simulink library "SCR"  (R2025b)
settings: Solver=VariableStepAuto  StartTime=0.0  StopTime=10.0  RelTol=1e-3
libraries: slpidlib x4
settings Model: Creator=Michael  LastModifiedBy=Michael

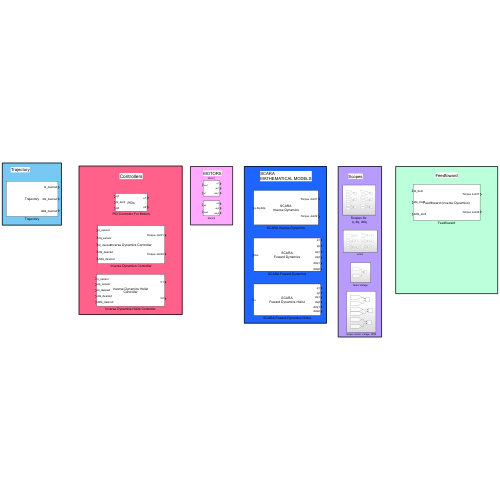
[thumbnail: Simulink's stored preview of the top-level diagram]
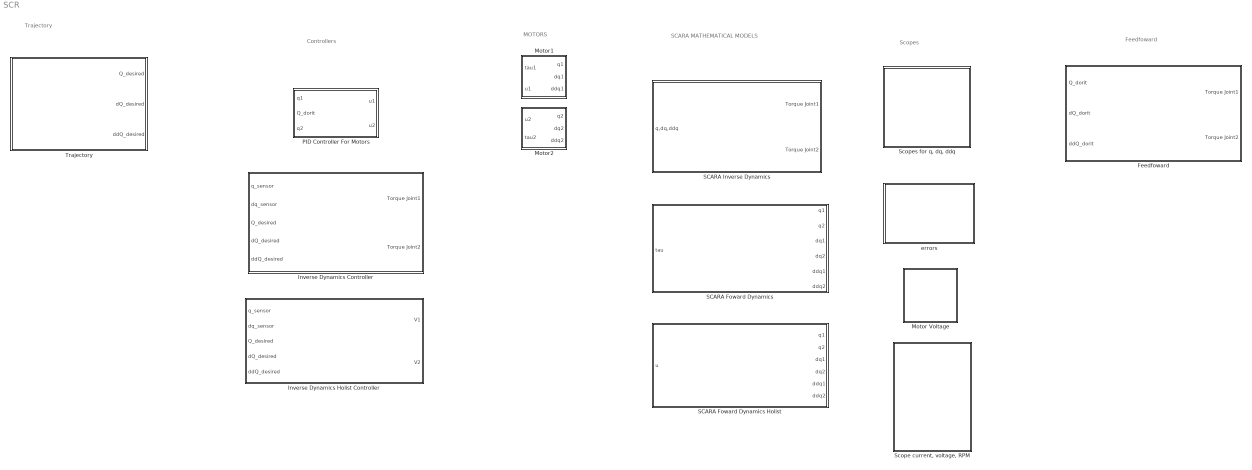
== system SCR ==
  note: MOTORS
  note: SCARA
      | MATHEMATICAL MODELS
  note: Scopes
  note: Trajectory
  note: Controllers
  note: Feedfoward
  Feedfoward : Subsystem
      mask Display: disp("Feedfoward (Inverse Dynamics)")
  Inverse Dynamics Controller : Subsystem
      mask Display: disp("Inverse Dynamics Controller")
  Inverse Dynamics Holist Controller : Subsystem
      mask Display:
      | disp("Inverse Dynamics Holist\n")
      | disp("\nController")
  Motor Voltage : Subsystem
  Motor1 : Subsystem
  Motor2 : Subsystem
  PID Controller For Motors : Subsystem
      mask Display: disp("PIDs")
  SCARA Foward Dynamics : Subsystem
      mask Display:
      | disp("SCARA\n")
      | disp("\nFoward Dynamics")
  SCARA Foward Dynamics Holist : Subsystem
      mask Display:
      | disp("SCARA\n")
      | disp("\nFoward Dynamics Holist")
  SCARA Inverse Dynamics : Subsystem
      mask Display:
      | disp("SCARA\n")
      | disp("\nInverse Dynamics")
  "Scope current, voltage, RPM" : Subsystem
  "Scopes for q, dq, ddq" : Subsystem
  Trajectory : Subsystem
      mask Display: disp("Trajectory")
  errors : Subsystem

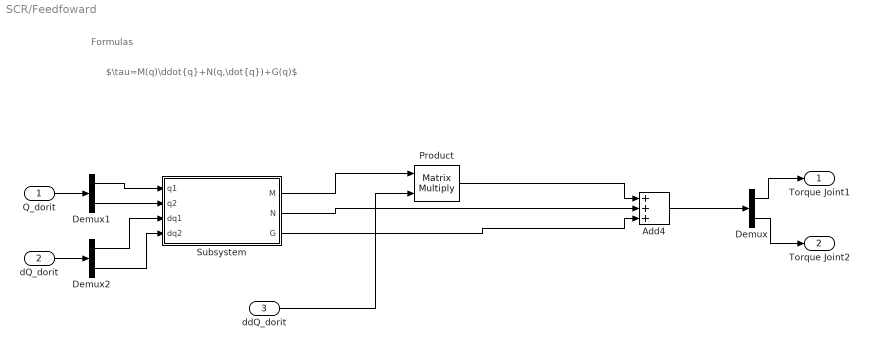
== system SCR/Feedfoward ==
  note: Formulas
  note: $\tau=M(q)\ddot{q}​+N(q,\dot{q})+G(q)$
  Q_dorit : Inport
  dQ_dorit : Inport  Port=2
  ddQ_dorit : Inport  Port=3
  Add4 : Sum  Inputs=+++
  Demux : Demux  Outputs=2
  Demux1 : Demux  Outputs=2
  Demux2 : Demux  Outputs=2
  Product : Product  Multiplication=Matrix(*)
  Subsystem : Subsystem
      mask Display: disp("Tau Components")
  Torque Joint1 : Outport
  Torque Joint2 : Outport  Port=2
  wires:
  Product/1 -> Add4/1
  Add4/1 -> Demux/1
  Demux/2 -> Torque Joint2/1
  Demux/1 -> Torque Joint1/1
  Subsystem/3(G) -> Add4/3
  Subsystem/1(M) -> Product/1
  Subsystem/2(N) -> Add4/2
  Q_dorit/1 -> Demux1/1
  Demux1/1 -> Subsystem/1(q1)
  Demux1/2 -> Subsystem/2(q2)
  dQ_dorit/1 -> Demux2/1
  Demux2/1 -> Subsystem/3(dq1)
  Demux2/2 -> Subsystem/4(dq2)
  ddQ_dorit/1 -> Product/2

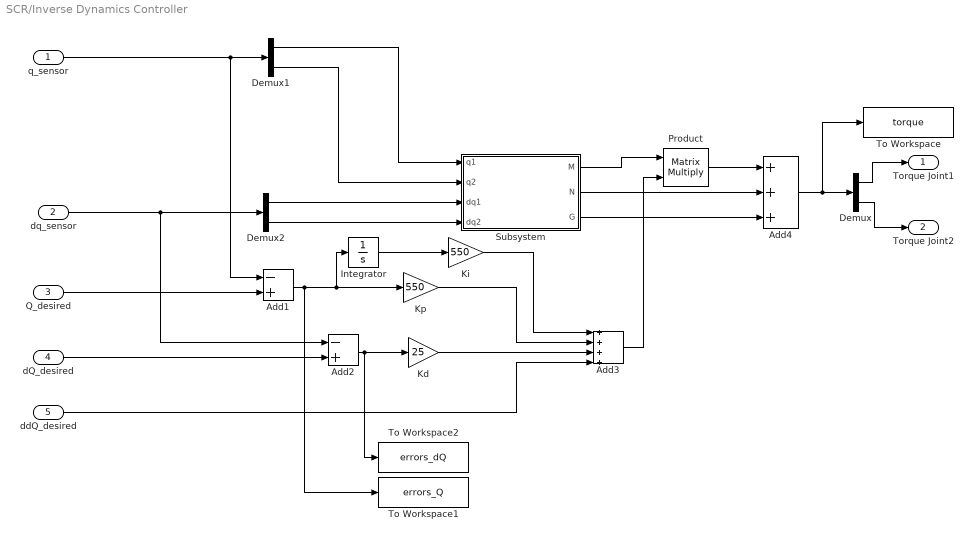
== system SCR/Inverse Dynamics Controller ==
  q_sensor : Inport
  dq_sensor : Inport  Port=2
  Q_desired : Inport  Port=3
  dQ_desired : Inport  Port=4
  ddQ_desired : Inport  Port=5
  Add1 : Sum  Inputs=-+
  Add2 : Sum  Inputs=-+
  Add3 : Sum  Inputs=++++
  Add4 : Sum  Inputs=+++
  Demux : Demux  Outputs=2
  Demux1 : Demux  Outputs=2
  Demux2 : Demux  Outputs=2
  Integrator : Integrator
  Kd : Gain  Gain=25
  Ki : Gain  Gain=550
  Kp : Gain  Gain=550
  Product : Product  Multiplication=Matrix(*)
  Subsystem : Subsystem
      mask Display: disp("Tau Components")
  To Workspace : ToWorkspace  VariableName=torque  SaveFormat=Timeseries  SampleTime=-1
  To Workspace1 : ToWorkspace  VariableName=errors_Q  SaveFormat=Timeseries  SampleTime=-1
  To Workspace2 : ToWorkspace  VariableName=errors_dQ  SaveFormat=Timeseries  SampleTime=-1
  Torque Joint1 : Outport
  Torque Joint2 : Outport  Port=2
  wires:
  Demux1/2 -> Subsystem/2(q2)
  dQ_desired/1 -> Add2/2
  Add1/1 -> Kp/1, Integrator/1, To Workspace1/1
  Add2/1 -> Kd/1, To Workspace2/1
  Add3/1 -> Product/2
  Add4/1 -> To Workspace/1, Demux/1
  Demux/2 -> Torque Joint2/1
  Demux/1 -> Torque Joint1/1
  Q_desired/1 -> Add1/2
  q_sensor/1 -> Add1/1, Demux1/1
  dq_sensor/1 -> Add2/1, Demux2/1
  Subsystem/1(M) -> Product/1
  Demux2/1 -> Subsystem/3(dq1)
  Demux2/2 -> Subsystem/4(dq2)
  Subsystem/2(N) -> Add4/2
  Demux1/1 -> Subsystem/1(q1)
  ddQ_desired/1 -> Add3/4
  Kd/1 -> Add3/3
  Kp/1 -> Add3/2
  Ki/1 -> Add3/1
  Integrator/1 -> Ki/1
  Subsystem/3(G) -> Add4/3
  Product/1 -> Add4/1

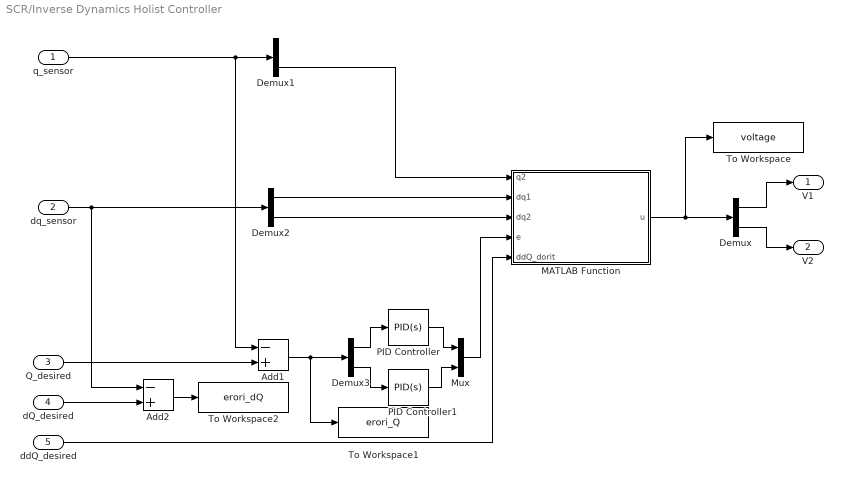
== system SCR/Inverse Dynamics Holist Controller ==
  q_sensor : Inport
  dq_sensor : Inport  Port=2
  Q_desired : Inport  Port=3
  dQ_desired : Inport  Port=4
  ddQ_desired : Inport  Port=5
  Add1 : Sum  Inputs=-+
  Add2 : Sum  Inputs=-+
  Demux{,1..3} (4 alike) : Demux  Outputs=2
  MATLAB Function : MATLAB Function  TreatAsAtomicUnit=on
  Mux : Mux  Inputs=2
  PID Controller : slpidlib/PID Controller  Controller=PID  Form=Parallel  TimeDomain=Continuous-time  UseExternalTs=off  SampleTime=-1  IntegratorMethod=Forward Euler  FilterMethod=Forward Euler  ControllerParametersSource=internal  P=14.7787089689118  I=5.05842239486125  UseKiTs=off  D=9.92816544136059  UseExternalDerivativeSource=off  N=1142.8279760416  UseFilter=on  TunerSelectOption=Transfer Function Based (PID Tuner App)  InitialConditionSource=internal  InitialConditionForIntegrator=0  InitialConditionForFilter=0  DifferentiatorICPrevScaledInput=0  ExternalReset=none  TrackingMode=off  Kt=1  LimitOutput=off  SatLimitsSource=internal  UpperSaturationLimit=0  LowerSaturationLimit=0  LinearizeAsGain=on  AntiWindupMode=none  Kb=1  LimitIntegrator=off  UpperIntegratorSaturationLimit=inf  LowerIntegratorSaturationLimit=-inf  POutMin=[]  POutMax=[]  IOutMin=[]  IOutMax=[]  DOutMin=[]  DOutMax=[]  NOutMin=[]  NOutMax=[]  SumOutMin=[]  SumOutMax=[]  SaturationOutMin=[]  SaturationOutMax=[]  PParamMin=[]  PParamMax=[]  IParamMin=[]  IParamMax=[]  DParamMin=[]  DParamMax=[]  NParamMin=[]  NParamMax=[]  KbParamMin=[]  KbParamMax=[]  KtParamMin=[]  KtParamMax=[]  KbOutMin=[]  KbOutMax=[]  KtOutMin=[]  KtOutMax=[]  IntegratorOutMin=[]  IntegratorOutMax=[]  FilterOutMin=[]  FilterOutMax=[]  SumI1OutMin=[]  SumI1OutMax=[]  SumI2OutMin=[]  SumI2OutMax=[]  SumI3OutMin=[]  SumI3OutMax=[]  SumI4OutMin=[]  SumI4OutMax=[]  SumDOutMin=[]  SumDOutMax=[]  DifferentiatorOutMin=[]  DifferentiatorOutMax=[]  FilterDiffOutCoefMin=[]  FilterDiffOutCoefMax=[]  ReciprocalOutMin=[]  ReciprocalOutMax=[]  SumDenOutMin=[]  SumDenOutMax=[]  SumNumOutMin=[]  SumNumOutMax=[]  DivideOutMin=[]  DivideOutMax=[]  UdiffTsProdOutMin=[]  UdiffTsProdOutMax=[]  NTsProdOutMin=[]  NTsProdOutMax=[]  UintegralTsProdOutMin=[]  UintegralTsProdOutMax=[]  UngainTsProdOutMin=[]  UngainTsProdOutMax=[]  ClampingZeroOutDataTypeStr=Inherit: Inherit via back propagation  ClampingZeroOutMin=[]  ClampingZeroOutMax=[]  FilterDenConstantOutDataTypeStr=Inherit: Inherit via back propagation  FilterDenConstantOutMin=[]  FilterDenConstantOutMax=[]  PCopyOutDataTypeStr=Inherit: Inherit via back propagation  PCopyOutMin=[]  PCopyOutMax=[]  NCopyOutDataTypeStr=Inherit: Inherit via back propagation  NCopyOutMin=[]  NCopyOutMax=[]  IntegratorContinuousStateAttributes=''  IntegratorStateMustResolveToSignalObject=off  IntegratorRTWStateStorageClass=Auto  FilterContinuousStateAttributes=''  FilterStateMustResolveToSignalObject=off  FilterRTWStateStorageClass=Auto  ParallelPVariant=InternalParameters  IdealPVariant=Disabled  IVariant=InternalParameters  DVariant=InternalParameters  IntegratorVariant=Continuous  SatVariant=Disabled  AWVariant=Passthrough  PCopyVariant=Disabled  TRVariant=Disabled  FdbkBlocksVariant=Forward  IdealPFdbkVariant=Disabled  SatFdbkVariant=Disabled  DerivativeFilterVariant=ContFilter  NVariant=InternalParameters  NCopyVariant=Disabled  FilterICVariant=InternalICsFilter  IntegratorICVariant=InternalICs  ExternalResetVariant=Disabled  TRSumVariant=Passthrough  SumFdbkVariant=Disabled  SumVariant=Sum_PID  TsampFilterVariant=InternalTs  TsampNgainVariant=Passthrough  TsampIntegralVariant=Disabled_SignalSpec  ExternalSaturationOutDataTypeStr=Inherit: Same as second input  DerivativeSourceVariant=ErrorSignal  PreIntVariant=InternalPreInt
  PID Controller1 : slpidlib/PID Controller  Controller=PID  Form=Parallel  TimeDomain=Continuous-time  UseExternalTs=off  SampleTime=-1  IntegratorMethod=Forward Euler  FilterMethod=Forward Euler  ControllerParametersSource=internal  P=16.3330424592972  I=6.55014962380407  UseKiTs=off  D=9.91721708236017  UseExternalDerivativeSource=off  N=1142.8279760416  UseFilter=on  TunerSelectOption=Transfer Function Based (PID Tuner App)  InitialConditionSource=internal  InitialConditionForIntegrator=0  InitialConditionForFilter=0  DifferentiatorICPrevScaledInput=0  ExternalReset=none  TrackingMode=off  Kt=1  LimitOutput=off  SatLimitsSource=internal  UpperSaturationLimit=24  LowerSaturationLimit=-24  LinearizeAsGain=on  AntiWindupMode=none  Kb=1  LimitIntegrator=off  UpperIntegratorSaturationLimit=inf  LowerIntegratorSaturationLimit=-inf  POutMin=[]  POutMax=[]  IOutMin=[]  IOutMax=[]  DOutMin=[]  DOutMax=[]  NOutMin=[]  NOutMax=[]  SumOutMin=[]  SumOutMax=[]  SaturationOutMin=[]  SaturationOutMax=[]  PParamMin=[]  PParamMax=[]  IParamMin=[]  IParamMax=[]  DParamMin=[]  DParamMax=[]  NParamMin=[]  NParamMax=[]  KbParamMin=[]  KbParamMax=[]  KtParamMin=[]  KtParamMax=[]  KbOutMin=[]  KbOutMax=[]  KtOutMin=[]  KtOutMax=[]  IntegratorOutMin=[]  IntegratorOutMax=[]  FilterOutMin=[]  FilterOutMax=[]  SumI1OutMin=[]  SumI1OutMax=[]  SumI2OutMin=[]  SumI2OutMax=[]  SumI3OutMin=[]  SumI3OutMax=[]  SumI4OutMin=[]  SumI4OutMax=[]  SumDOutMin=[]  SumDOutMax=[]  DifferentiatorOutMin=[]  DifferentiatorOutMax=[]  FilterDiffOutCoefMin=[]  FilterDiffOutCoefMax=[]  ReciprocalOutMin=[]  ReciprocalOutMax=[]  SumDenOutMin=[]  SumDenOutMax=[]  SumNumOutMin=[]  SumNumOutMax=[]  DivideOutMin=[]  DivideOutMax=[]  UdiffTsProdOutMin=[]  UdiffTsProdOutMax=[]  NTsProdOutMin=[]  NTsProdOutMax=[]  UintegralTsProdOutMin=[]  UintegralTsProdOutMax=[]  UngainTsProdOutMin=[]  UngainTsProdOutMax=[]  ClampingZeroOutDataTypeStr=Inherit: Inherit via back propagation  ClampingZeroOutMin=[]  ClampingZeroOutMax=[]  FilterDenConstantOutDataTypeStr=Inherit: Inherit via back propagation  FilterDenConstantOutMin=[]  FilterDenConstantOutMax=[]  PCopyOutDataTypeStr=Inherit: Inherit via back propagation  PCopyOutMin=[]  PCopyOutMax=[]  NCopyOutDataTypeStr=Inherit: Inherit via back propagation  NCopyOutMin=[]  NCopyOutMax=[]  IntegratorContinuousStateAttributes=''  IntegratorStateMustResolveToSignalObject=off  IntegratorRTWStateStorageClass=Auto  FilterContinuousStateAttributes=''  FilterStateMustResolveToSignalObject=off  FilterRTWStateStorageClass=Auto  ParallelPVariant=InternalParameters  IdealPVariant=Disabled  IVariant=InternalParameters  DVariant=InternalParameters  IntegratorVariant=Continuous  SatVariant=Disabled  AWVariant=Passthrough  PCopyVariant=Disabled  TRVariant=Disabled  FdbkBlocksVariant=Forward  IdealPFdbkVariant=Disabled  SatFdbkVariant=Disabled  DerivativeFilterVariant=ContFilter  NVariant=InternalParameters  NCopyVariant=Disabled  FilterICVariant=InternalICsFilter  IntegratorICVariant=InternalICs  ExternalResetVariant=Disabled  TRSumVariant=Passthrough  SumFdbkVariant=Disabled  SumVariant=Sum_PID  TsampFilterVariant=InternalTs  TsampNgainVariant=Passthrough  TsampIntegralVariant=Disabled_SignalSpec  ExternalSaturationOutDataTypeStr=Inherit: Same as second input  DerivativeSourceVariant=ErrorSignal  PreIntVariant=InternalPreInt
  To Workspace : ToWorkspace  VariableName=voltage  SaveFormat=Timeseries  SampleTime=-1
  To Workspace1 : ToWorkspace  VariableName=erori_Q  SaveFormat=Timeseries  SampleTime=-1
  To Workspace2 : ToWorkspace  VariableName=erori_dQ  SaveFormat=Timeseries  SampleTime=-1
  V1 : Outport
  V2 : Outport  Port=2
  wires:
  Demux2/1 -> MATLAB Function/2(dq1)
  Demux1/2 -> MATLAB Function/1(q2)
  Mux/1 -> MATLAB Function/4(e)
  PID Controller1/1 -> Mux/2
  PID Controller/1 -> Mux/1
  Demux3/2 -> PID Controller1/1
  Demux3/1 -> PID Controller/1
  Add1/1 -> To Workspace1/1, Demux3/1
  MATLAB Function/1(u) -> To Workspace/1, Demux/1
  ddQ_desired/1 -> MATLAB Function/5(ddQ_dorit)
  Demux2/2 -> MATLAB Function/3(dq2)
  dq_sensor/1 -> Add2/1, Demux2/1
  q_sensor/1 -> Demux1/1, Add1/1
  Q_desired/1 -> Add1/2
  Demux/1 -> V1/1
  Demux/2 -> V2/1
  dQ_desired/1 -> Add2/2
  Add2/1 -> To Workspace2/1

== system SCR/Motor Voltage ==
  motorTorques : Scope  NumInputPorts=2
      settings: DataLoggingVariableName=ScopeData6
  wires:
  [u1] -> motorTorques/1
  [u2] -> motorTorques/2

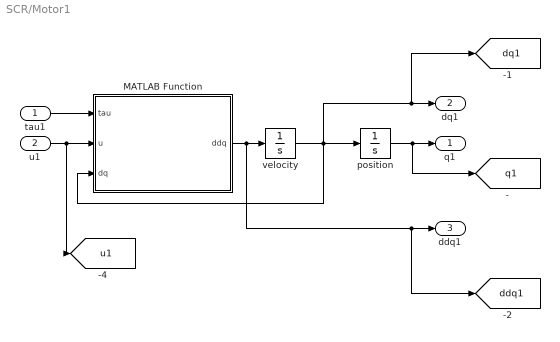
== system SCR/Motor1 ==
  tau1 : Inport
  u1 : Inport  Port=2
  MATLAB Function : MATLAB Function  TreatAsAtomicUnit=on
  position : Integrator
  velocity : Integrator
  q1 : Outport
  dq1 : Outport  Port=2
  ddq1 : Outport  Port=3
  tag scope: ddq1=global, dq1=global, q1=global, u1=global
  wires:
  MATLAB Function/1(ddq) -> [ddq1], ddq1/1, velocity/1
  u1/1 -> [u1], MATLAB Function/2(u)
  tau1/1 -> MATLAB Function/1(tau)
  velocity/1 -> [dq1], dq1/1, MATLAB Function/3(dq), position/1
  position/1 -> [q1], q1/1

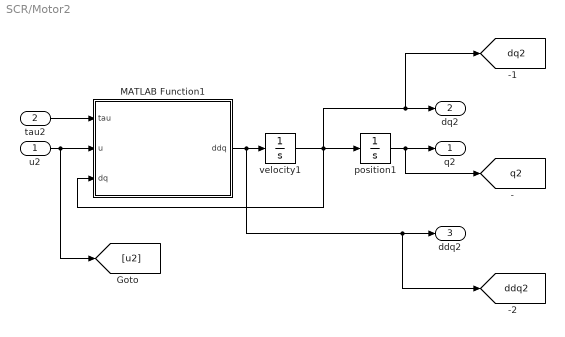
== system SCR/Motor2 ==
  u2 : Inport
  tau2 : Inport  Port=2
  MATLAB Function1 : MATLAB Function  TreatAsAtomicUnit=on
  position1 : Integrator
  velocity1 : Integrator
  q2 : Outport
  dq2 : Outport  Port=2
  ddq2 : Outport  Port=3
  tag scope: ddq2=global, dq2=global, q2=global
  wires:
  MATLAB Function1/1(ddq) -> [ddq2], ddq2/1, velocity1/1
  velocity1/1 -> [dq2], dq2/1, MATLAB Function1/3(dq), position1/1
  tau2/1 -> MATLAB Function1/1(tau)
  position1/1 -> [q2], q2/1
  u2/1 -> [u2], MATLAB Function1/2(u)

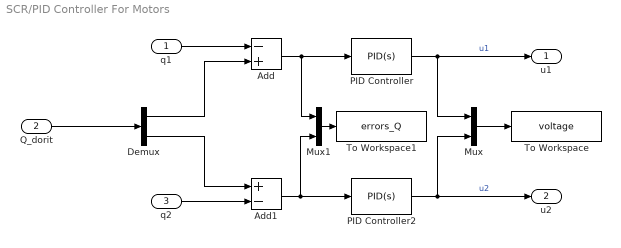
== system SCR/PID Controller For Motors ==
  q1 : Inport
  Q_dorit : Inport  Port=2
  q2 : Inport  Port=3
  Add : Sum  Inputs=-+
  Add1 : Sum  Inputs=+-
  Demux : Demux  Outputs=2
  Mux : Mux  Inputs=2
  Mux1 : Mux  Inputs=2
  PID Controller : slpidlib/PID Controller  Controller=PID  Form=Parallel  TimeDomain=Continuous-time  UseExternalTs=off  SampleTime=-1  IntegratorMethod=Forward Euler  FilterMethod=Forward Euler  ControllerParametersSource=internal  P=17042.9277196606  I=696153.474275857  UseKiTs=off  D=-7.42275649016862  UseExternalDerivativeSource=off  N=2296.03756262702  UseFilter=on  TunerSelectOption=Transfer Function Based (PID Tuner App)  InitialConditionSource=internal  InitialConditionForIntegrator=0  InitialConditionForFilter=0  DifferentiatorICPrevScaledInput=0  ExternalReset=none  TrackingMode=off  Kt=1  LimitOutput=on  SatLimitsSource=internal  UpperSaturationLimit=24  LowerSaturationLimit=-24  LinearizeAsGain=off  AntiWindupMode=clamping  Kb=10  LimitIntegrator=off  UpperIntegratorSaturationLimit=inf  LowerIntegratorSaturationLimit=-inf  POutMin=[]  POutMax=[]  IOutMin=[]  IOutMax=[]  DOutMin=[]  DOutMax=[]  NOutMin=[]  NOutMax=[]  SumOutMin=[]  SumOutMax=[]  SaturationOutMin=[]  SaturationOutMax=[]  PParamMin=[]  PParamMax=[]  IParamMin=[]  IParamMax=[]  DParamMin=[]  DParamMax=[]  NParamMin=[]  NParamMax=[]  KbParamMin=[]  KbParamMax=[]  KtParamMin=[]  KtParamMax=[]  KbOutMin=[]  KbOutMax=[]  KtOutMin=[]  KtOutMax=[]  IntegratorOutMin=[]  IntegratorOutMax=[]  FilterOutMin=[]  FilterOutMax=[]  SumI1OutMin=[]  SumI1OutMax=[]  SumI2OutMin=[]  SumI2OutMax=[]  SumI3OutMin=[]  SumI3OutMax=[]  SumI4OutMin=[]  SumI4OutMax=[]  SumDOutMin=[]  SumDOutMax=[]  DifferentiatorOutMin=[]  DifferentiatorOutMax=[]  FilterDiffOutCoefMin=[]  FilterDiffOutCoefMax=[]  ReciprocalOutMin=[]  ReciprocalOutMax=[]  SumDenOutMin=[]  SumDenOutMax=[]  SumNumOutMin=[]  SumNumOutMax=[]  DivideOutMin=[]  DivideOutMax=[]  UdiffTsProdOutMin=[]  UdiffTsProdOutMax=[]  NTsProdOutMin=[]  NTsProdOutMax=[]  UintegralTsProdOutMin=[]  UintegralTsProdOutMax=[]  UngainTsProdOutMin=[]  UngainTsProdOutMax=[]  ClampingZeroOutDataTypeStr=Inherit: Inherit via back propagation  ClampingZeroOutMin=[]  ClampingZeroOutMax=[]  FilterDenConstantOutDataTypeStr=Inherit: Inherit via back propagation  FilterDenConstantOutMin=[]  FilterDenConstantOutMax=[]  PCopyOutDataTypeStr=Inherit: Inherit via back propagation  PCopyOutMin=[]  PCopyOutMax=[]  NCopyOutDataTypeStr=Inherit: Inherit via back propagation  NCopyOutMin=[]  NCopyOutMax=[]  IntegratorContinuousStateAttributes=''  IntegratorStateMustResolveToSignalObject=off  IntegratorRTWStateStorageClass=Auto  FilterContinuousStateAttributes=''  FilterStateMustResolveToSignalObject=off  FilterRTWStateStorageClass=Auto  ParallelPVariant=InternalParameters  IdealPVariant=Disabled  IVariant=InternalParameters  DVariant=InternalParameters  IntegratorVariant=Continuous  SatVariant=Enabled  AWVariant=ContClampingParallel  PCopyVariant=Disabled  TRVariant=Disabled  FdbkBlocksVariant=Forward  IdealPFdbkVariant=Disabled  SatFdbkVariant=Disabled  DerivativeFilterVariant=ContFilter  NVariant=InternalParameters  NCopyVariant=Disabled  FilterICVariant=InternalICsFilter  IntegratorICVariant=InternalICs  ExternalResetVariant=Disabled  TRSumVariant=Passthrough  SumFdbkVariant=Disabled  SumVariant=Sum_PID  TsampFilterVariant=InternalTs  TsampNgainVariant=Passthrough  TsampIntegralVariant=Disabled_SignalSpec  ExternalSaturationOutDataTypeStr=Inherit: Same as second input  DerivativeSourceVariant=ErrorSignal  PreIntVariant=InternalPreInt
  PID Controller2 : slpidlib/PID Controller  Controller=PID  Form=Parallel  TimeDomain=Continuous-time  UseExternalTs=off  SampleTime=-1  IntegratorMethod=Forward Euler  FilterMethod=Forward Euler  ControllerParametersSource=internal  P=19726.0931917022  I=877163.671153983  UseKiTs=off  D=28.399075244163  UseExternalDerivativeSource=off  N=2735.67202823723  UseFilter=on  TunerSelectOption=Transfer Function Based (PID Tuner App)  InitialConditionSource=internal  InitialConditionForIntegrator=0  InitialConditionForFilter=0  DifferentiatorICPrevScaledInput=0  ExternalReset=none  TrackingMode=off  Kt=1  LimitOutput=on  SatLimitsSource=internal  UpperSaturationLimit=24  LowerSaturationLimit=-24  LinearizeAsGain=off  AntiWindupMode=clamping  Kb=10  LimitIntegrator=off  UpperIntegratorSaturationLimit=inf  LowerIntegratorSaturationLimit=-inf  POutMin=[]  POutMax=[]  IOutMin=[]  IOutMax=[]  DOutMin=[]  DOutMax=[]  NOutMin=[]  NOutMax=[]  SumOutMin=[]  SumOutMax=[]  SaturationOutMin=[]  SaturationOutMax=[]  PParamMin=[]  PParamMax=[]  IParamMin=[]  IParamMax=[]  DParamMin=[]  DParamMax=[]  NParamMin=[]  NParamMax=[]  KbParamMin=[]  KbParamMax=[]  KtParamMin=[]  KtParamMax=[]  KbOutMin=[]  KbOutMax=[]  KtOutMin=[]  KtOutMax=[]  IntegratorOutMin=[]  IntegratorOutMax=[]  FilterOutMin=[]  FilterOutMax=[]  SumI1OutMin=[]  SumI1OutMax=[]  SumI2OutMin=[]  SumI2OutMax=[]  SumI3OutMin=[]  SumI3OutMax=[]  SumI4OutMin=[]  SumI4OutMax=[]  SumDOutMin=[]  SumDOutMax=[]  DifferentiatorOutMin=[]  DifferentiatorOutMax=[]  FilterDiffOutCoefMin=[]  FilterDiffOutCoefMax=[]  ReciprocalOutMin=[]  ReciprocalOutMax=[]  SumDenOutMin=[]  SumDenOutMax=[]  SumNumOutMin=[]  SumNumOutMax=[]  DivideOutMin=[]  DivideOutMax=[]  UdiffTsProdOutMin=[]  UdiffTsProdOutMax=[]  NTsProdOutMin=[]  NTsProdOutMax=[]  UintegralTsProdOutMin=[]  UintegralTsProdOutMax=[]  UngainTsProdOutMin=[]  UngainTsProdOutMax=[]  ClampingZeroOutDataTypeStr=Inherit: Inherit via back propagation  ClampingZeroOutMin=[]  ClampingZeroOutMax=[]  FilterDenConstantOutDataTypeStr=Inherit: Inherit via back propagation  FilterDenConstantOutMin=[]  FilterDenConstantOutMax=[]  PCopyOutDataTypeStr=Inherit: Inherit via back propagation  PCopyOutMin=[]  PCopyOutMax=[]  NCopyOutDataTypeStr=Inherit: Inherit via back propagation  NCopyOutMin=[]  NCopyOutMax=[]  IntegratorContinuousStateAttributes=''  IntegratorStateMustResolveToSignalObject=off  IntegratorRTWStateStorageClass=Auto  FilterContinuousStateAttributes=''  FilterStateMustResolveToSignalObject=off  FilterRTWStateStorageClass=Auto  ParallelPVariant=InternalParameters  IdealPVariant=Disabled  IVariant=InternalParameters  DVariant=InternalParameters  IntegratorVariant=Continuous  SatVariant=Enabled  AWVariant=ContClampingParallel  PCopyVariant=Disabled  TRVariant=Disabled  FdbkBlocksVariant=Forward  IdealPFdbkVariant=Disabled  SatFdbkVariant=Disabled  DerivativeFilterVariant=ContFilter  NVariant=InternalParameters  NCopyVariant=Disabled  FilterICVariant=InternalICsFilter  IntegratorICVariant=InternalICs  ExternalResetVariant=Disabled  TRSumVariant=Passthrough  SumFdbkVariant=Disabled  SumVariant=Sum_PID  TsampFilterVariant=InternalTs  TsampNgainVariant=Passthrough  TsampIntegralVariant=Disabled_SignalSpec  ExternalSaturationOutDataTypeStr=Inherit: Same as second input  DerivativeSourceVariant=ErrorSignal  PreIntVariant=InternalPreInt
  To Workspace : ToWorkspace  VariableName=voltage  SaveFormat=Timeseries  SampleTime=-1
  To Workspace1 : ToWorkspace  VariableName=errors_Q  SaveFormat=Timeseries  SampleTime=-1
  u1 : Outport
  u2 : Outport  Port=2
  wires:
  Demux/2 -> Add1/1
  Demux/1 -> Add/2
  q1/1 -> Add/1
  Add/1 -> Mux1/1, PID Controller/1
  Q_dorit/1 -> Demux/1
  Add1/1 -> PID Controller2/1, Mux1/2
  q2/1 -> Add1/2
  PID Controller/1 -> Mux/1, u1/1  "u1"
  PID Controller2/1 -> Mux/2, u2/1  "u2"
  Mux/1 -> To Workspace/1
  Mux1/1 -> To Workspace1/1

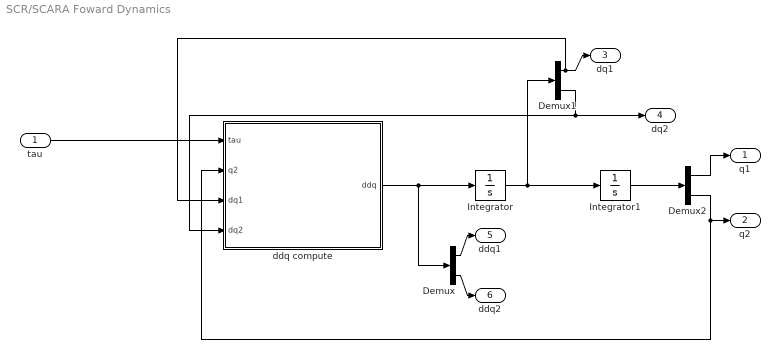
== system SCR/SCARA Foward Dynamics ==
  tau : Inport
  Demux : Demux  Outputs=2
  Demux1 : Demux  Outputs=2
  Demux2 : Demux  Outputs=2
  Integrator : Integrator
  Integrator1 : Integrator
  ddq compute : MATLAB Function  TreatAsAtomicUnit=on
  q1 : Outport
  q2 : Outport  Port=2
  dq1 : Outport  Port=3
  dq2 : Outport  Port=4
  ddq1 : Outport  Port=5
  ddq2 : Outport  Port=6
  wires:
  ddq compute/1(ddq) -> Integrator/1, Demux/1
  tau/1 -> ddq compute/1(tau)
  Integrator/1 -> Demux1/1, Integrator1/1
  Demux/1 -> ddq1/1
  Demux/2 -> ddq2/1
  Demux1/1 -> ddq compute/3(dq1), dq1/1
  Demux1/2 -> ddq compute/4(dq2), dq2/1
  Integrator1/1 -> Demux2/1
  Demux2/1 -> q1/1
  Demux2/2 -> ddq compute/2(q2), q2/1

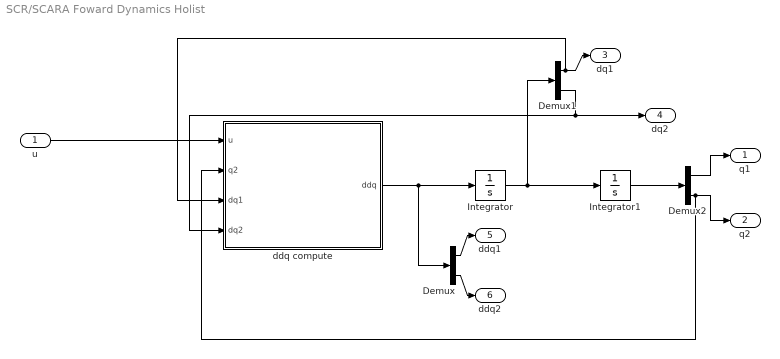
== system SCR/SCARA Foward Dynamics Holist ==
  u : Inport
  Demux : Demux  Outputs=2
  Demux1 : Demux  Outputs=2
  Demux2 : Demux  Outputs=2
  Integrator : Integrator
  Integrator1 : Integrator
  ddq compute : MATLAB Function  TreatAsAtomicUnit=on
  q1 : Outport
  q2 : Outport  Port=2
  dq1 : Outport  Port=3
  dq2 : Outport  Port=4
  ddq1 : Outport  Port=5
  ddq2 : Outport  Port=6
  wires:
  Demux2/2 -> q2/1, ddq compute/2(q2)
  Demux2/1 -> q1/1
  Integrator1/1 -> Demux2/1
  Demux1/2 -> dq2/1, ddq compute/4(dq2)
  Demux1/1 -> dq1/1, ddq compute/3(dq1)
  Demux/2 -> ddq2/1
  Demux/1 -> ddq1/1
  Integrator/1 -> Integrator1/1, Demux1/1
  u/1 -> ddq compute/1(u)
  ddq compute/1(ddq) -> Demux/1, Integrator/1

== system SCR/SCARA Inverse Dynamics ==
  q,dq,ddq : Inport
  Demux : Demux  Outputs=2
  Demux1 : Demux  Outputs=5
  Memory : Memory
  To Workspace : ToWorkspace  VariableName=torque  SaveFormat=Timeseries  SampleTime=-1
  tau compute : MATLAB Function  TreatAsAtomicUnit=on
  Torque Joint1 : Outport
  Torque Joint2 : Outport  Port=2
  wires:
  Memory/1 -> Demux1/1
  Demux1/5 -> tau compute/5(ddq2)
  Demux1/4 -> tau compute/4(dq2)
  Demux1/3 -> tau compute/3(q2)
  Demux1/2 -> tau compute/2(ddq1)
  Demux1/1 -> tau compute/1(dq1)
  q,dq,ddq/1 -> Memory/1
  Demux/1 -> Torque Joint1/1
  Demux/2 -> Torque Joint2/1
  tau compute/1(tau) -> To Workspace/1, Demux/1

== system SCR/Scope current, voltage, RPM ==
  Scope : Scope  NumInputPorts=2
      settings: DataLoggingVariableName=ScopeData7
  Scope1 : Scope  NumInputPorts=2
      settings: DataLoggingVariableName=ScopeData8
  Scope2 : Scope  NumInputPorts=2
      settings: DataLoggingVariableName=ScopeData9
  wires:
  [motorCurrent1] -> Scope/1
  [motorCurrent2] -> Scope/2
  [motorVoltage2] -> Scope1/2
  [motorVoltage1] -> Scope1/1
  [motorRPM1] -> Scope2/1
  [motorRPM2] -> Scope2/2

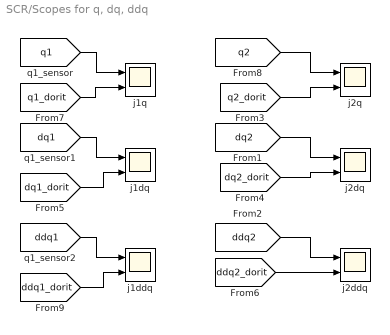
== system SCR/Scopes for q, dq, ddq ==
  j1ddq : Scope  NumInputPorts=2
      settings: ActiveDisplayYMinimum=-1.59649  ActiveDisplayYMaximum=10.27308  DataLoggingVariableName=ScopeData3
  j1dq : Scope  NumInputPorts=2
      settings: ActiveDisplayYMinimum=-1.59649  ActiveDisplayYMaximum=10.27308
  j1q : Scope  NumInputPorts=2
      settings: ActiveDisplayYMinimum=-1.59649  ActiveDisplayYMaximum=10.27308  DataLoggingVariableName=ScopeData5
  j2ddq : Scope  NumInputPorts=2
      settings: ActiveDisplayYMinimum=-0.26586  ActiveDisplayYMaximum=2.39277  DataLoggingVariableName=ScopeData4
  j2dq : Scope  NumInputPorts=2
      settings: ActiveDisplayYMinimum=-0.26586  ActiveDisplayYMaximum=2.39277  DataLoggingVariableName=ScopeData2
  j2q : Scope  NumInputPorts=2
      settings: ActiveDisplayYMinimum=-0.26586  ActiveDisplayYMaximum=2.39277
  wires:
  [dq1] -> j1dq/1
  [q2] -> j2q/1
  [q1] -> j1q/1
  [ddq2] -> j2ddq/1
  [ddq1] -> j1ddq/1
  [dq2] -> j2dq/1
  [dq1_dorit] -> j1dq/2
  [q1_dorit] -> j1q/2
  [ddq1_dorit] -> j1ddq/2
  [q2_dorit] -> j2q/2
  [ddq2_dorit] -> j2ddq/2
  [dq2_dorit] -> j2dq/2

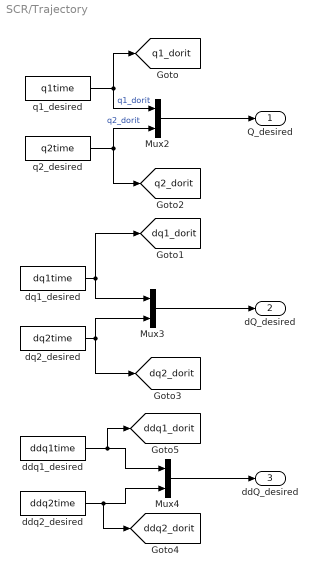
== system SCR/Trajectory ==
  Mux2 : Mux  Inputs=2
  Mux3 : Mux  Inputs=2
  Mux4 : Mux  Inputs=2
  ddq1_desired : FromWorkspace  VariableName=ddq1time
  ddq2_desired : FromWorkspace  VariableName=ddq2time
  dq1_desired : FromWorkspace  VariableName=dq1time
  dq2_desired : FromWorkspace  VariableName=dq2time
  q1_desired : FromWorkspace  VariableName=q1time
  q2_desired : FromWorkspace  VariableName=q2time
  Q_desired : Outport
  dQ_desired : Outport  Port=2
  ddQ_desired : Outport  Port=3
  tag scope: ddq1_dorit=global, ddq2_dorit=global, dq1_dorit=global, dq2_dorit=global, q1_dorit=global, q2_dorit=global
  wires:
  Mux4/1 -> ddQ_desired/1
  Mux2/1 -> Q_desired/1
  Mux3/1 -> dQ_desired/1
  q2_desired/1 -> Mux2/2, [q2_dorit]  "q2_dorit"
  q1_desired/1 -> Mux2/1, [q1_dorit]  "q1_dorit"
  dq1_desired/1 -> [dq1_dorit], Mux3/1
  dq2_desired/1 -> Mux3/2, [dq2_dorit]
  ddq1_desired/1 -> [ddq1_dorit], Mux4/1
  ddq2_desired/1 -> [ddq2_dorit], Mux4/2

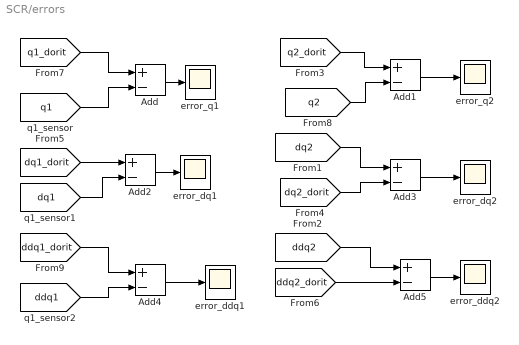
== system SCR/errors ==
  Add{,1..5} (6 alike) : Sum  Inputs=+-
  error_ddq1 : Scope
      settings: ActiveDisplayYMinimum=-1.59649  ActiveDisplayYMaximum=10.27308  DataLoggingVariableName=ScopeData2
  error_ddq2 : Scope
      settings: ActiveDisplayYMinimum=-1.59649  ActiveDisplayYMaximum=10.27308  DataLoggingVariableName=ScopeData5
  error_dq1 : Scope
      settings: ActiveDisplayYMinimum=-1.59649  ActiveDisplayYMaximum=10.27308  DataLoggingVariableName=ScopeData3
  error_dq2 : Scope
      settings: ActiveDisplayYMinimum=-0.26586  ActiveDisplayYMaximum=2.39277  DataLoggingVariableName=ScopeData6
  error_q1 : Scope
      settings: ActiveDisplayYMinimum=-1.59649  ActiveDisplayYMaximum=10.27308  DataLoggingVariableName=ScopeData4
  error_q2 : Scope
      settings: ActiveDisplayYMinimum=-0.26586  ActiveDisplayYMaximum=2.39277  DataLoggingVariableName=ScopeData7
  wires:
  [ddq2] -> Add5/1
  [ddq2_dorit] -> Add5/2
  Add/1 -> error_q1/1
  [q1_dorit] -> Add/1
  [q1] -> Add/2
  [q2_dorit] -> Add1/1
  [q2] -> Add1/2
  Add1/1 -> error_q2/1
  [dq1_dorit] -> Add2/1
  Add2/1 -> error_dq1/1
  [dq1] -> Add2/2
  Add3/1 -> error_dq2/1
  [dq2] -> Add3/1
  [dq2_dorit] -> Add3/2
  [ddq1_dorit] -> Add4/1
  [ddq1] -> Add4/2
  Add4/1 -> error_ddq1/1
  Add5/1 -> error_ddq2/1

== system SCR/Feedfoward/Subsystem ==
  q1 : Inport
  q2 : Inport  Port=2
  dq1 : Inport  Port=3
  dq2 : Inport  Port=4
  MATLAB Function1 : MATLAB Function  TreatAsAtomicUnit=on
  MATLAB Function2 : MATLAB Function  TreatAsAtomicUnit=on
  MATLAB Function3 : MATLAB Function  TreatAsAtomicUnit=on
  M : Outport
  N : Outport  Port=2
  G : Outport  Port=3
  wires:
  MATLAB Function3/1(M) -> M/1
  MATLAB Function1/1(N) -> N/1
  q2/1 -> MATLAB Function2/2(q2), MATLAB Function1/1(q2), MATLAB Function3/1(q2)
  dq2/1 -> MATLAB Function1/3(dq2)
  dq1/1 -> MATLAB Function1/2(dq1)
  MATLAB Function2/1(G) -> G/1
  q1/1 -> MATLAB Function2/1(q1)

== system SCR/Inverse Dynamics Controller/Subsystem ==
  q1 : Inport
  q2 : Inport  Port=2
  dq1 : Inport  Port=3
  dq2 : Inport  Port=4
  MATLAB Function1 : MATLAB Function  TreatAsAtomicUnit=on
  MATLAB Function2 : MATLAB Function  TreatAsAtomicUnit=on
  MATLAB Function3 : MATLAB Function  TreatAsAtomicUnit=on
  M : Outport
  N : Outport  Port=2
  G : Outport  Port=3
  wires:
  MATLAB Function3/1(M) -> M/1
  MATLAB Function1/1(N) -> N/1
  q2/1 -> MATLAB Function2/2(q2), MATLAB Function1/1(q2), MATLAB Function3/1(q2)
  dq2/1 -> MATLAB Function1/3(dq2)
  dq1/1 -> MATLAB Function1/2(dq1)
  MATLAB Function2/1(G) -> G/1
  q1/1 -> MATLAB Function2/1(q1)

== matlab function SCR/Inverse Dynamics Holist Controller/MATLAB Function ==
  data: u output; q2 input; dq1 input; dq2 input; e input; ddQ_dorit input
function u = inverseDynamicsControl(q2, dq1, dq2, e, ddQ_dorit)
    % parameters of SCARA
    m1 = 1;      
    m2 = 2;      
    l1 = 0.2;
    lc2 = 0.1;
    lc1 = 0.1;
    Izz1 = 3.68e-3;
    Izz2 = 7.366e-3;

    % parameters motor
    J_t = 72.8e-6;
    i_r = 103;
    n = 1/1.74;
    b = 0.1;
    k_M = 27.3e-3;
    R = 0.108;

    factor1 = diag(1/(n*i_r^2));
    factor2 = diag(b + k_M^2/R);
    factor3 = diag(k_M/(i_r*R));
    factor4 = inv(diag(k_M/(i_r*R)));
    

    M = factor4  * (diag(J_t) + factor1 * [m2*l1^2 + 2*m2*cos(q2)*l1*lc2 + m1*lc1^2 + m2*lc2^2 + Izz1 + Izz2, m2*lc2^2 + l1*m2*cos(q2)*lc2 + Izz2; 
     m2*lc2^2 + l1*m2*cos(q2)*lc2 + Izz2, m2*lc2^2 + Izz2]);


    % coriolis
    B_coriolis = [-2*l1*lc2*m2*sin(q2);
         0];

    
    % centrifugal
    Cn = [0, -l1*lc2*m2*sin(q2);
          l1*lc2*m2*sin(q2), 0];


    N = Cn*[dq1^2; dq2^2] + B_coriolis*dq1*dq2;
    N = factor4 * factor1 * N;

    B = factor4 * factor2;
    B = B * [dq1; dq2];
    
    % gravitational
    G = [0;0];

    u = M*(e+ddQ_dorit) + B + N;

== matlab function SCR/SCARA Foward Dynamics Holist/ddq compute ==
  data: u input; ddq output; q2 input; dq1 input; dq2 input
function ddq = foward_dynamics(u, q2, dq1, dq2)
    % parameters SCARA
    m1 = 1;      
    m2 = 2;      
    l1 = 0.2;
    lc2 = 0.1;
    lc1 = 0.1;
    Izz1 = 3.68e-3;
    Izz2 = 7.366e-3;
    
    % parameters motor+gearing
    J_t = 72.8e-6;
    i_r = 103;
    n = 1/1.74;
    b = 0.1;
    k_M = 27.3e-3;
    R = 0.108;


    factor1 = diag(1/(n*i_r^2));
    factor2 = diag(b + k_M^2/R);
    factor3 = diag(1/(n*i_r^2));
    factor4 = diag(k_M/(i_r*R));

    % mass inertia
    M = diag(J_t) +  factor1 * [m2*l1^2 + 2*m2*cos(q2)*l1*lc2 + m1*lc1^2 + m2*lc2^2 + Izz1 + Izz2, m2*lc2^2 + l1*m2*cos(q2)*lc2 + Izz2; 
     m2*lc2^2 + l1*m2*cos(q2)*lc2 + Izz2, m2*lc2^2 + Izz2];

     % coriolis
    B_coriolis = [-2*l1*lc2*m2*sin(q2);
         0];
    
    % centrifugal
    Cn = [0, -l1*lc2*m2*sin(q2);
          l1*lc2*m2*sin(q2), 0];
    % coriolis + centrifugal
    N = Cn*[dq1^2; dq2^2] + B_coriolis*dq1*dq2;

    N = factor3 * N;
    
    % comanda
    u = factor4 * u;

    B = factor2 * [dq1; dq2];
    
    % gravitationalul
    G = [0;0];

    ddq = inv(M) * (u - N - B - G);

== matlab function SCR/Feedfoward/Subsystem/MATLAB Function1 ==
  data: N output; q2 input; dq1 input; dq2 input
function N = velocityProductTorque(q2, dq1, dq2)
 
    m2 = 1.6;      
    l1 = 0.18;
    lc2 = 0.09;


    % coriolis
    B = [-2*l1*lc2*m2*sin(q2);
         0];
    velocity_vector = dq1*dq2;
    
    % centrifugal
    Cn = [0, -l1*lc2*m2*sin(q2);
          l1*lc2*m2*sin(q2), 0];
    velocity_vector_squared = [dq1^2; dq2^2];
    

    N = Cn*velocity_vector_squared + B*velocity_vector;
end

== matlab function SCR/Feedfoward/Subsystem/MATLAB Function2 ==
  data: q1 input; G output; q2 input
function G = gravity(q1, q2)

    
    m1 = 1.6;      
    m2 = 1.6;        
    l1 = 0.18;
    lc1 = 0.09;
    lc2 = 0.09;
    g = 9.82;
    
    G = [0;0];

end

== matlab function SCR/Inverse Dynamics Controller/Subsystem/MATLAB Function1 ==
  data: N output; q2 input; dq1 input; dq2 input
function N = velocityProductTorque(q2, dq1, dq2)
 
    m2 = 1.6;      
    l1 = 0.18;
    lc2 = 0.09;

    % coriolis
    B = [-2*l1*lc2*m2*sin(q2);
         0];
    
    % centrifugal
    Cn = [0, -l1*lc2*m2*sin(q2);
          l1*lc2*m2*sin(q2), 0]; 

    N = Cn*[dq1^2; dq2^2]; + B*[dq1*dq2];
end

== matlab function SCR/Inverse Dynamics Controller/Subsystem/MATLAB Function2 ==
  data: q1 input; G output; q2 input
function G = gravity(q1, q2)

    
    m1 = 1.6;      
    m2 = 1.6;        
    l1 = 0.18;
    lc1 = 0.09;
    lc2 = 0.09;
    g = 9.82;
    
    G = [0;0];

end

== matlab function SCR/Inverse Dynamics Controller/Subsystem/MATLAB Function3 ==
  data: q2 input; M output
function M = massInertia(q2)

    m1 = 1.6;      
    m2 = 1.6;      
    l1 = 0.18;
    lc2 = 0.09;
    lc1 = 0.09;
    Izz1 = 0.05;
    Izz2 = 0.05;

    M = [m2*l1^2 + 2*m2*cos(q2)*l1*lc2 + m1*lc1^2 + m2*lc2^2 + Izz1 + Izz2, m2*lc2^2 + l1*m2*cos(q2)*lc2 + Izz2; 
     m2*lc2^2 + l1*m2*cos(q2)*lc2 + Izz2, m2*lc2^2 + Izz2];
end

== matlab function SCR/Feedfoward/Subsystem/MATLAB Function3 ==
  data: q2 input; M output
function M = massInertia(q2)

    m1 = 1.6;      
    m2 = 1.6;      
    l1 = 0.18;
    lc2 = 0.09;
    lc1 = 0.09;
    Izz1 = 0.05;
    Izz2 = 0.05;

    M = [m2*l1^2 + 2*m2*cos(q2)*l1*lc2 + m1*lc1^2 + m2*lc2^2 + Izz1 + Izz2, m2*lc2^2 + l1*m2*cos(q2)*lc2 + Izz2; 
     m2*lc2^2 + l1*m2*cos(q2)*lc2 + Izz2, m2*lc2^2 + Izz2];
end

== matlab function SCR/SCARA Inverse Dynamics/tau compute ==
  data: dq1 input; ddq1 input; q2 input; tau output; dq2 input; ddq2 input
function tau = tau_compute(dq1, ddq1, q2, dq2, ddq2)
    
    % parameters SCARA
    m1 = 1;      
    m2 = 2;      
    l1 = 0.2;
    lc2 = 0.1;
    lc1 = 0.1;
    Izz1 = 3.68e-3;
    Izz2 = 7.366e-3;
   
    % mass inertia
    M = [m2*l1^2 + 2*m2*cos(q2)*l1*lc2 + m1*lc1^2 + m2*lc2^2 + Izz1 + Izz2, m2*lc2^2 + l1*m2*cos(q2)*lc2 + Izz2; 
     m2*lc2^2 + l1*m2*cos(q2)*lc2 + Izz2, m2*lc2^2 + Izz2];
    M = M * [ddq1; ddq2];

     % coriolis
    B_coriolis = [-2*l1*lc2*m2*sin(q2);
         0];
    
    % centrifugal
    Cn = [0, -l1*lc2*m2*sin(q2);
          l1*lc2*m2*sin(q2), 0];
    % coriolis + centrifugal
    N = Cn*[dq1^2; dq2^2] + B_coriolis*dq1*dq2;

    G = [0;0];

    tau = M + N + G;

== matlab function SCR/SCARA Foward Dynamics/ddq compute ==
  data: tau input; ddq output; q2 input; dq1 input; dq2 input
function ddq = foward_dynamics(tau, q2, dq1, dq2)
    m1 = 1;      
    m2 = 2;      
    l1 = 0.2;
    lc2 = 0.1;
    lc1 = 0.1;
    Izz1 = 3.68e-3;
    Izz2 = 7.366e-3;

    % mass inertia
    M = [m2*l1^2 + 2*m2*cos(q2)*l1*lc2 + m1*lc1^2 + m2*lc2^2 + Izz1 + Izz2, m2*lc2^2 + l1*m2*cos(q2)*lc2 + Izz2; 
     m2*lc2^2 + l1*m2*cos(q2)*lc2 + Izz2, m2*lc2^2 + Izz2];

     % coriolis
    B = [-2*l1*lc2*m2*sin(q2);
         0];
    
    % centrifugal
    Cn = [0, -l1*lc2*m2*sin(q2);
          l1*lc2*m2*sin(q2), 0];

    N = Cn*[dq1^2; dq2^2] + B*dq1*dq2;

    G = [0;0];

    ddq = inv(M) * (tau - N - G);

== matlab function SCR/Motor1/MATLAB Function ==
  data: tau input; ddq output; u input; dq input
function ddq = Motor(tau, u, dq)

    % parameters of the motor + gearing
    
    b = 0.1; %[Nms/rad]
    k_M = 27.3*10^-3; %[mNm/A]
    randament = 1/1.74; 
    i_r = 103;
    R = 0.200; %[ohm]
    J_a = 72.8*10^-6; %[gcm^2]


    factor1 = (b + k_M^2/R)*dq;
    factor2 = tau/(randament*i_r^2);
    factor3 = k_M / (i_r * R) * u;
    ddq = 1/J_a * (factor3 - factor1 - factor2);

== matlab function SCR/Motor2/MATLAB Function1 ==
  data: tau input; ddq output; u input; dq input
function ddq = Motor(tau, u, dq)

    % parameters of the motor+gearing
    
    b = 0.1; %[Nms/rad]
    k_M = 27.3*10^-3; %[mNm/A]
    randament = 1/1.74; 
    i_r = 103;
    R = 0.200; %[ohm]
    J_a = 72.8*10^-6; %[gcm^2]


    factor1 = (b + k_M^2/R)*dq;
    factor2 = tau/(randament*i_r^2);
    factor3 = k_M / (i_r * R) * u;
    ddq = 1/J_a * (factor3 - factor1 - factor2);
